simulink model "I2S"  (R2023b)
settings: Solver=VariableStepAuto  StartTime=0.0  StopTime=1  RelTol=1e-3
values from neighbouring files (symbols this model uses):
  cnt1_LRCLK = 511    [DATA_GEN.m]
  cnt2_SCLK = 7    [DATA_GEN.m]
libraries: hdlsllib x8
settings Model: Creator=31651  LastModifiedBy=31651

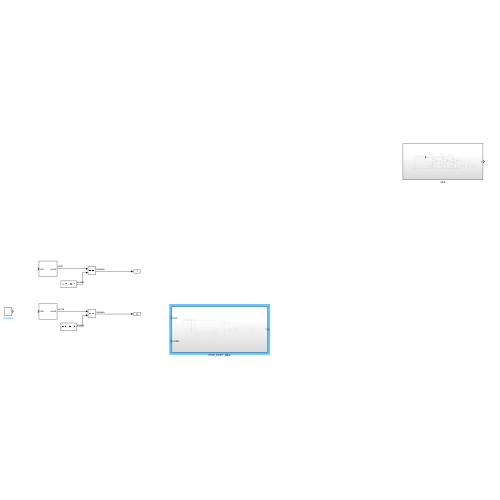
[thumbnail: Simulink's stored preview of the top-level diagram]
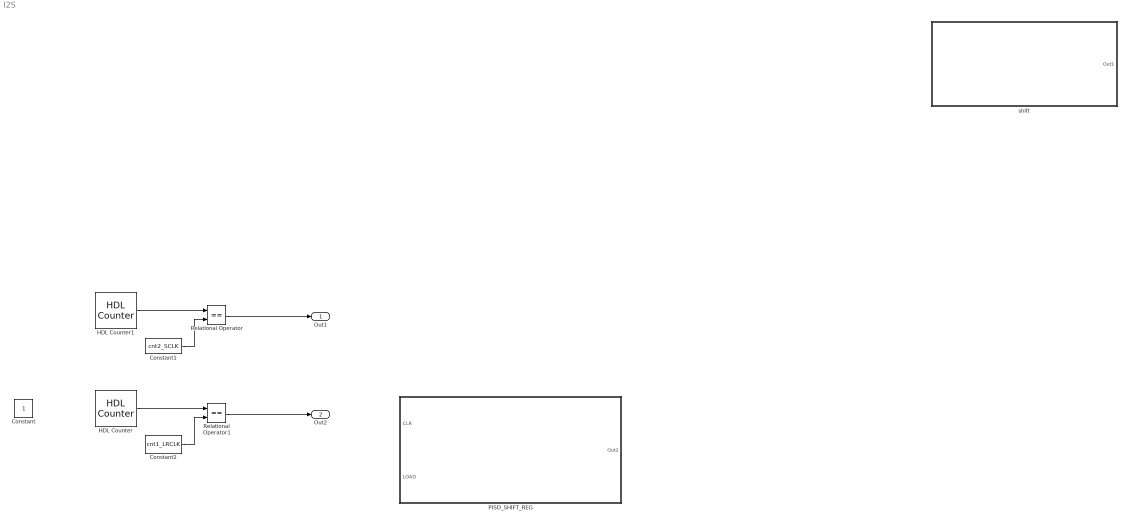
== system I2S ==
  Constant : Constant  OutDataTypeStr=boolean  SampleTime=1
  Constant1 : Constant  Value=cnt2_SCLK
  Constant2 : Constant  Value=cnt1_LRCLK
  HDL Counter : hdlsllib/Sources/HDL Counter  CountType=Count limited  CountInit=0  CountStep=1  CountMax=cnt1_LRCLK  CountFromType=Initial value  CountFrom=0  CountResetPort=off  CountLoadPort=off  CountEnbPort=on  CountDirPort=off  CountHitOutputPort=off  CountDataType=Unsigned  CountWordLen=16  CountFracLen=0  CountSampTime=1
  HDL Counter1 : hdlsllib/Sources/HDL Counter  CountType=Count limited  CountInit=0  CountStep=1  CountMax=cnt2_SCLK  CountFromType=Initial value  CountFrom=0  CountResetPort=off  CountLoadPort=off  CountEnbPort=on  CountDirPort=off  CountHitOutputPort=off  CountDataType=Unsigned  CountWordLen=8  CountFracLen=0  CountSampTime=1
  PISO_SHIFT_REG : Subsystem
  Relational Operator : RelationalOperator  Operator===  OutDataTypeStr=boolean  InputSameDT=off
  Relational Operator1 : RelationalOperator  Operator===  OutDataTypeStr=boolean  InputSameDT=off
  shift : Subsystem
  Out1 : Outport  VectorParamsAs1DForOutWhenUnconnected=off
  Out2 : Outport  Port=2  VectorParamsAs1DForOutWhenUnconnected=off
  wires:
  HDL Counter1/1 -> Relational Operator/1
  Constant1/1 -> Relational Operator/2
  Constant2/1 -> Relational Operator1/2
  HDL Counter/1 -> Relational Operator1/1
  Relational Operator/1 -> Out1/1
  Relational Operator1/1 -> Out2/1

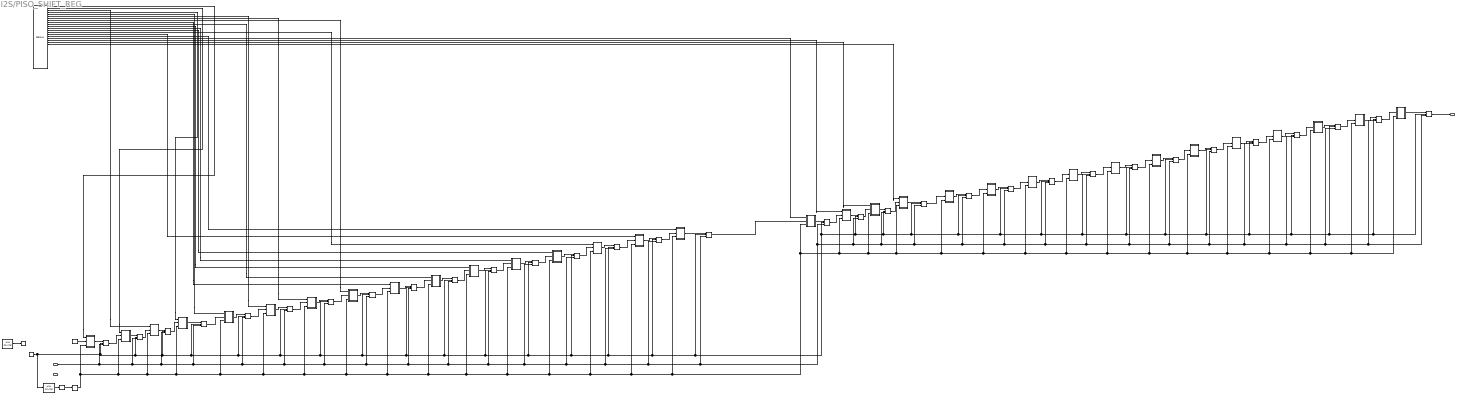
== system I2S/PISO_SHIFT_REG ==
  note: LOAD=0写入数据
      | LOAD=1 移位
  CLR : Inport
  LOAD : Inport  Port=2
  CLK : Constant  OutDataTypeStr=boolean  SampleTime=1/1000
  Compare To Constant : hdlsllib/Logic and Bit Operations/Compare To Constant  relop=>=  const=50  OutDataTypeStr=boolean
  Compare To Constant1 : hdlsllib/Logic and Bit Operations/Compare To Constant  relop=>=  const=10  OutDataTypeStr=boolean
  Constant5 : Constant  Value=0  OutDataTypeStr=boolean  SampleTime=1
  Delay{,1..15,17..24,26..33} (32 alike) : Delay  DelayLength=1  ExternalReset=Either  ShowEnablePort=on
      settings: InputPortMap=u0,e6,r5
  Delay16 : Delay  DelayLength=1  InitialCondition=0
  Demux : Demux  Outputs=32
      settings: DisplayOption=none
  HDL Counter : hdlsllib/Sources/HDL Counter  CountType=Count limited  CountInit=0  CountStep=1  CountMax=25  CountFromType=Initial value  CountFrom=0  CountResetPort=off  CountLoadPort=off  CountEnbPort=off  CountDirPort=off  CountHitOutputPort=off  CountDataType=Unsigned  CountWordLen=8  CountFracLen=0  CountSampTime=1
  HDL Counter1 : hdlsllib/Sources/HDL Counter  CountType=Count limited  CountInit=0  CountStep=1  CountMax=500  CountFromType=Initial value  CountFrom=0  CountResetPort=off  CountLoadPort=off  CountEnbPort=on  CountDirPort=off  CountHitOutputPort=off  CountDataType=Unsigned  CountWordLen=16  CountFracLen=0  CountSampTime=1
  MUX : Subsystem
  MUX1 : Subsystem
  MUX10 : Subsystem
  MUX11 : Subsystem
  MUX12 : Subsystem
  MUX13 : Subsystem
  MUX14 : Subsystem
  MUX15 : Subsystem
  MUX16 : Subsystem
  MUX17 : Subsystem
  MUX18 : Subsystem
  MUX19 : Subsystem
  MUX2 : Subsystem
  MUX20 : Subsystem
  MUX21 : Subsystem
  MUX22 : Subsystem
  MUX23 : Subsystem
  MUX24 : Subsystem
  MUX25 : Subsystem
  MUX26 : Subsystem
  MUX27 : Subsystem
  MUX28 : Subsystem
  MUX29 : Subsystem
  MUX3 : Subsystem
  MUX30 : Subsystem
  MUX31 : Subsystem
  MUX4 : Subsystem
  MUX5 : Subsystem
  MUX6 : Subsystem
  MUX7 : Subsystem
  MUX8 : Subsystem
  MUX9 : Subsystem
  Out2 : Outport  VectorParamsAs1DForOutWhenUnconnected=off
  wires:
  MUX/1(Out1) -> Delay/1
  Demux/2 -> MUX1/1(In1)
  MUX1/1(Out1) -> Delay1/1
  Delay/1 -> MUX1/2(In2)
  MUX2/1(Out1) -> Delay2/1
  Demux/3 -> MUX2/1(In1)
  Delay1/1 -> MUX2/2(In2)
  Demux/4 -> MUX3/1(In1)
  Delay2/1 -> MUX3/2(In2)
  MUX3/1(Out1) -> Delay3/1
  Constant5/1 -> MUX/2(In2)
  Demux/1 -> MUX/1(In1)
  MUX4/1(Out1) -> Delay4/1
  MUX5/1(Out1) -> Delay5/1
  MUX6/1(Out1) -> Delay6/1
  Delay3/1 -> MUX4/2(In2)
  Delay4/1 -> MUX5/2(In2)
  Delay5/1 -> MUX6/2(In2)
  Delay8/1 -> MUX9/2(In2)
  Delay7/1 -> MUX8/2(In2)
  MUX8/1(Out1) -> Delay8/1
  MUX9/1(Out1) -> Delay9/1
  MUX7/1(Out1) -> Delay7/1
  Delay11/1 -> MUX12/2(In2)
  Delay10/1 -> MUX11/2(In2)
  MUX11/1(Out1) -> Delay11/1
  MUX12/1(Out1) -> Delay12/1
  MUX10/1(Out1) -> Delay10/1
  Delay14/1 -> MUX15/2(In2)
  Delay13/1 -> MUX14/2(In2)
  MUX14/1(Out1) -> Delay14/1
  MUX15/1(Out1) -> Delay15/1
  MUX13/1(Out1) -> Delay13/1
  Delay6/1 -> MUX7/2(In2)
  Delay9/1 -> MUX10/2(In2)
  Delay12/1 -> MUX13/2(In2)
  Demux/5 -> MUX4/1(In1)
  Demux/6 -> MUX5/1(In1)
  Demux/7 -> MUX6/1(In1)
  Demux/8 -> MUX7/1(In1)
  Demux/9 -> MUX8/1(In1)
  Demux/10 -> MUX9/1(In1)
  Demux/11 -> MUX10/1(In1)
  Demux/12 -> MUX11/1(In1)
  Demux/13 -> MUX12/1(In1)
  Demux/14 -> MUX13/1(In1)
  Demux/15 -> MUX14/1(In1)
  Demux/16 -> MUX15/1(In1)
  HDL Counter/1 -> Compare To Constant/1
  Compare To Constant1/1 -> Delay16/1
  HDL Counter1/1 -> Compare To Constant1/1
  ? -> MUX21/1(In1)
  CLK/1 -> HDL Counter1/1, Delay1/2, Delay2/2, Delay8/2, Delay10/2, Delay11/2, Delay12/2, Delay13/2, Delay14/2, Delay15/2, Delay17/2, Delay18/2, Delay26/2, Delay32/2, Delay19/2, Delay20/2, Delay21/2, Delay22/2, Delay23/2, Delay24/2, Delay33/2, Delay31/2, Delay30/2, Delay29/2, Delay28/2, Delay27/2, Delay9/2, Delay7/2, Delay6/2, Delay5/2, Delay4/2, Delay3/2, Delay/2
  ? -> MUX29/1(In1)
  ? -> MUX19/1(In1)
  ? -> MUX18/1(In1)
  Delay26/1 -> MUX25/2(In2)
  MUX25/1(Out1) -> Delay27/1
  Delay16/1 -> MUX/3(SEL), MUX1/3(SEL), MUX4/3(SEL), MUX5/3(SEL), MUX6/3(SEL), MUX7/3(SEL), MUX8/3(SEL), MUX9/3(SEL), MUX10/3(SEL), MUX11/3(SEL), MUX12/3(SEL), MUX13/3(SEL), MUX14/3(SEL), MUX15/3(SEL), MUX16/3(SEL), MUX17/3(SEL), MUX26/3(SEL), MUX27/3(SEL), MUX28/3(SEL), MUX29/3(SEL), MUX30/3(SEL), MUX31/3(SEL), MUX18/3(SEL), MUX19/3(SEL), MUX20/3(SEL), MUX21/3(SEL), MUX22/3(SEL), MUX23/3(SEL), MUX25/3(SEL), MUX24/3(SEL), MUX3/3(SEL), MUX2/3(SEL)
  MUX31/1(Out1) -> Delay33/1
  MUX29/1(Out1) -> Delay31/1
  MUX30/1(Out1) -> Delay32/1
  Delay31/1 -> MUX30/2(In2)
  Delay32/1 -> MUX31/2(In2)
  MUX17/1(Out1) -> Delay18/1
  Delay17/1 -> MUX17/2(In2)
  MUX16/1(Out1) -> Delay17/1
  ? -> MUX28/1(In1)
  Delay29/1 -> MUX28/2(In2)
  Delay28/1 -> MUX27/2(In2)
  ? -> MUX27/1(In1)
  MUX27/1(Out1) -> Delay29/1
  Delay21/1 -> MUX21/2(In2)
  MUX20/1(Out1) -> Delay21/1
  ? -> MUX31/1(In1)
  Delay24/1 -> Out2/1
  Demux/20 -> MUX25/1(In1)
  CLR/1 -> Delay/3, Delay24/3, Delay23/3, Delay22/3, Delay21/3, Delay20/3, Delay19/3, Delay33/3, Delay32/3, Delay31/3, Delay30/3, Delay29/3, Delay28/3, Delay27/3, Delay26/3, Delay18/3, Delay17/3, Delay15/3, Delay14/3, Delay13/3, Delay12/3, Delay11/3, Delay10/3, Delay9/3, Delay8/3, Delay7/3, Delay6/3, Delay5/3, Delay4/3, Delay3/3, Delay2/3, Delay1/3
  ? -> MUX20/1(In1)
  Demux/18 -> MUX17/1(In1)
  Demux/17 -> MUX16/1(In1)
  Delay18/1 -> MUX24/2(In2)
  ? -> MUX26/1(In1)
  ? -> MUX22/1(In1)
  ? -> MUX30/1(In1)
  Delay27/1 -> MUX26/2(In2)
  MUX26/1(Out1) -> Delay28/1
  Delay20/1 -> MUX20/2(In2)
  MUX18/1(Out1) -> Delay19/1
  Delay19/1 -> MUX19/2(In2)
  MUX28/1(Out1) -> Delay30/1
  MUX23/1(Out1) -> Delay24/1
  Delay15/1 -> MUX16/2(In2)
  Delay33/1 -> MUX18/2(In2)
  Delay22/1 -> MUX22/2(In2)
  Delay23/1 -> MUX23/2(In2)
  ? -> MUX23/1(In1)
  MUX21/1(Out1) -> Delay22/1
  MUX24/1(Out1) -> Delay26/1
  Delay30/1 -> MUX29/2(In2)
  MUX19/1(Out1) -> Delay20/1
  MUX22/1(Out1) -> Delay23/1
  Demux/19 -> MUX24/1(In1)

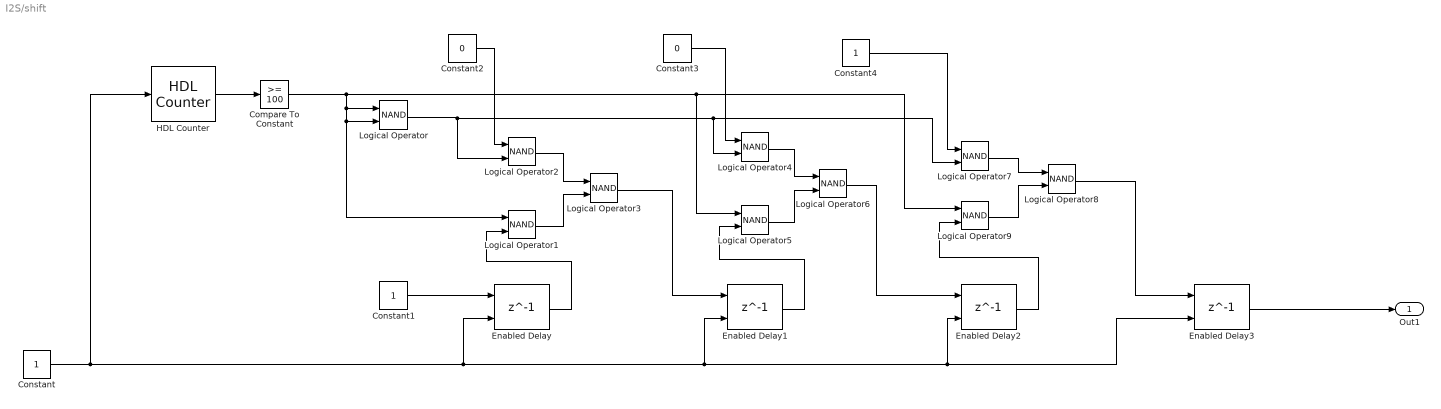
== system I2S/shift ==
  Compare To Constant : hdlsllib/Logic and Bit Operations/Compare To Constant  relop=>=  const=100  OutDataTypeStr=boolean
  Constant : Constant  OutDataTypeStr=boolean  SampleTime=1
  Constant1 : Constant  OutDataTypeStr=boolean  SampleTime=1
  Constant2 : Constant  Value=0  OutDataTypeStr=boolean  SampleTime=1
  Constant3 : Constant  Value=0  OutDataTypeStr=boolean  SampleTime=1
  Constant4 : Constant  OutDataTypeStr=boolean  SampleTime=1
  Enabled Delay{,1..3} (4 alike) : Delay  DelayLength=1  ShowEnablePort=on
      settings: InputPortMap=u0,e6
  HDL Counter : hdlsllib/Sources/HDL Counter  CountType=Count limited  CountInit=0  CountStep=1  CountMax=1000  CountFromType=Initial value  CountFrom=0  CountResetPort=off  CountLoadPort=off  CountEnbPort=on  CountDirPort=off  CountHitOutputPort=off  CountDataType=Unsigned  CountWordLen=16  CountFracLen=0  CountSampTime=1
  Logical Operator{,1..9} (10 alike) : Logic  Operator=NAND  AllPortsSameDT=off  OutDataTypeStr=boolean
  Out1 : Outport  VectorParamsAs1DForOutWhenUnconnected=off
  wires:
  Logical Operator1/1 -> Logical Operator3/2
  Logical Operator2/1 -> Logical Operator3/1
  Logical Operator/1 -> Logical Operator2/2, Logical Operator7/2, Logical Operator4/2
  Enabled Delay/1 -> Logical Operator1/2
  Compare To Constant/1 -> Logical Operator9/1, Logical Operator5/1, Logical Operator1/1, Logical Operator/2, Logical Operator/1
  Logical Operator5/1 -> Logical Operator6/2
  Logical Operator4/1 -> Logical Operator6/1
  Logical Operator3/1 -> Enabled Delay1/1
  Enabled Delay1/1 -> Logical Operator5/2
  Logical Operator7/1 -> Logical Operator8/1
  Logical Operator9/1 -> Logical Operator8/2
  Enabled Delay2/1 -> Logical Operator9/2
  Logical Operator6/1 -> Enabled Delay2/1
  Logical Operator8/1 -> Enabled Delay3/1
  Constant/1 -> HDL Counter/1, Enabled Delay/2, Enabled Delay1/2, Enabled Delay3/2, Enabled Delay2/2
  Constant2/1 -> Logical Operator2/1
  Constant3/1 -> Logical Operator4/1
  Constant4/1 -> Logical Operator7/1
  Enabled Delay3/1 -> Out1/1
  Constant1/1 -> Enabled Delay/1
  HDL Counter/1 -> Compare To Constant/1

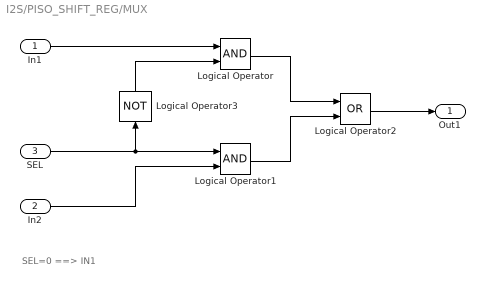
== system I2S/PISO_SHIFT_REG/MUX ==
  note: SEL=0 ==> IN1
  In1 : Inport
  In2 : Inport  Port=2
  SEL : Inport  Port=3  OutDataTypeStr=boolean
  Logical Operator : Logic  AllPortsSameDT=off  OutDataTypeStr=boolean
  Logical Operator1 : Logic  AllPortsSameDT=off  OutDataTypeStr=boolean
  Logical Operator2 : Logic  Operator=OR  AllPortsSameDT=off  OutDataTypeStr=boolean
  Logical Operator3 : Logic  Operator=NOT  AllPortsSameDT=off  OutDataTypeStr=boolean
  Out1 : Outport  VectorParamsAs1DForOutWhenUnconnected=off
  wires:
  In1/1 -> Logical Operator/1
  SEL/1 -> Logical Operator3/1, Logical Operator1/1
  Logical Operator3/1 -> Logical Operator/2
  Logical Operator1/1 -> Logical Operator2/2
  Logical Operator/1 -> Logical Operator2/1
  Logical Operator2/1 -> Out1/1
  In2/1 -> Logical Operator1/2

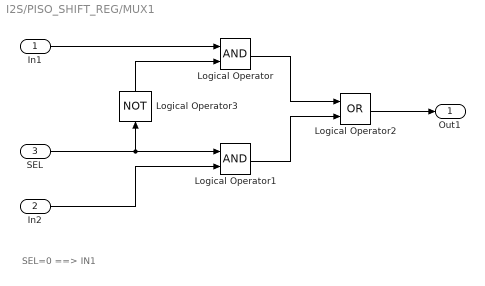
== system I2S/PISO_SHIFT_REG/MUX1 ==
  note: SEL=0 ==> IN1
  In1 : Inport
  In2 : Inport  Port=2
  SEL : Inport  Port=3  OutDataTypeStr=boolean
  Logical Operator : Logic  AllPortsSameDT=off  OutDataTypeStr=boolean
  Logical Operator1 : Logic  AllPortsSameDT=off  OutDataTypeStr=boolean
  Logical Operator2 : Logic  Operator=OR  AllPortsSameDT=off  OutDataTypeStr=boolean
  Logical Operator3 : Logic  Operator=NOT  AllPortsSameDT=off  OutDataTypeStr=boolean
  Out1 : Outport  VectorParamsAs1DForOutWhenUnconnected=off
  wires:
  In1/1 -> Logical Operator/1
  SEL/1 -> Logical Operator3/1, Logical Operator1/1
  Logical Operator3/1 -> Logical Operator/2
  Logical Operator1/1 -> Logical Operator2/2
  Logical Operator/1 -> Logical Operator2/1
  Logical Operator2/1 -> Out1/1
  In2/1 -> Logical Operator1/2

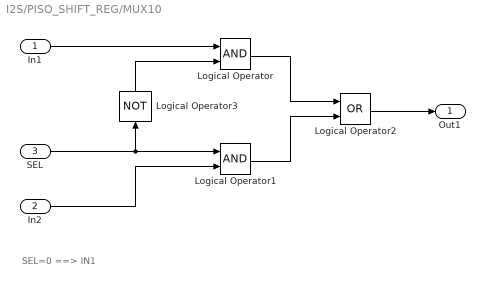
== system I2S/PISO_SHIFT_REG/MUX10 ==
  note: SEL=0 ==> IN1
  In1 : Inport
  In2 : Inport  Port=2
  SEL : Inport  Port=3  OutDataTypeStr=boolean
  Logical Operator : Logic  AllPortsSameDT=off  OutDataTypeStr=boolean
  Logical Operator1 : Logic  AllPortsSameDT=off  OutDataTypeStr=boolean
  Logical Operator2 : Logic  Operator=OR  AllPortsSameDT=off  OutDataTypeStr=boolean
  Logical Operator3 : Logic  Operator=NOT  AllPortsSameDT=off  OutDataTypeStr=boolean
  Out1 : Outport  VectorParamsAs1DForOutWhenUnconnected=off
  wires:
  In1/1 -> Logical Operator/1
  SEL/1 -> Logical Operator3/1, Logical Operator1/1
  Logical Operator3/1 -> Logical Operator/2
  Logical Operator1/1 -> Logical Operator2/2
  Logical Operator/1 -> Logical Operator2/1
  Logical Operator2/1 -> Out1/1
  In2/1 -> Logical Operator1/2

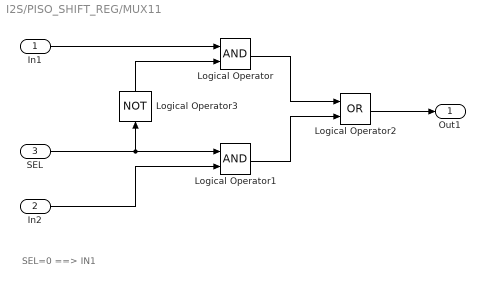
== system I2S/PISO_SHIFT_REG/MUX11 ==
  note: SEL=0 ==> IN1
  In1 : Inport
  In2 : Inport  Port=2
  SEL : Inport  Port=3  OutDataTypeStr=boolean
  Logical Operator : Logic  AllPortsSameDT=off  OutDataTypeStr=boolean
  Logical Operator1 : Logic  AllPortsSameDT=off  OutDataTypeStr=boolean
  Logical Operator2 : Logic  Operator=OR  AllPortsSameDT=off  OutDataTypeStr=boolean
  Logical Operator3 : Logic  Operator=NOT  AllPortsSameDT=off  OutDataTypeStr=boolean
  Out1 : Outport  VectorParamsAs1DForOutWhenUnconnected=off
  wires:
  In1/1 -> Logical Operator/1
  SEL/1 -> Logical Operator3/1, Logical Operator1/1
  Logical Operator3/1 -> Logical Operator/2
  Logical Operator1/1 -> Logical Operator2/2
  Logical Operator/1 -> Logical Operator2/1
  Logical Operator2/1 -> Out1/1
  In2/1 -> Logical Operator1/2

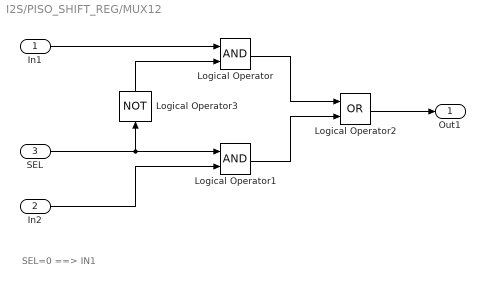
== system I2S/PISO_SHIFT_REG/MUX12 ==
  note: SEL=0 ==> IN1
  In1 : Inport
  In2 : Inport  Port=2
  SEL : Inport  Port=3  OutDataTypeStr=boolean
  Logical Operator : Logic  AllPortsSameDT=off  OutDataTypeStr=boolean
  Logical Operator1 : Logic  AllPortsSameDT=off  OutDataTypeStr=boolean
  Logical Operator2 : Logic  Operator=OR  AllPortsSameDT=off  OutDataTypeStr=boolean
  Logical Operator3 : Logic  Operator=NOT  AllPortsSameDT=off  OutDataTypeStr=boolean
  Out1 : Outport  VectorParamsAs1DForOutWhenUnconnected=off
  wires:
  In1/1 -> Logical Operator/1
  SEL/1 -> Logical Operator3/1, Logical Operator1/1
  Logical Operator3/1 -> Logical Operator/2
  Logical Operator1/1 -> Logical Operator2/2
  Logical Operator/1 -> Logical Operator2/1
  Logical Operator2/1 -> Out1/1
  In2/1 -> Logical Operator1/2

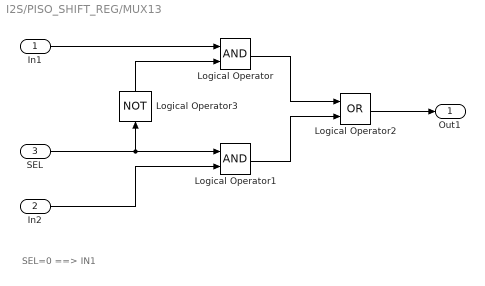
== system I2S/PISO_SHIFT_REG/MUX13 ==
  note: SEL=0 ==> IN1
  In1 : Inport
  In2 : Inport  Port=2
  SEL : Inport  Port=3  OutDataTypeStr=boolean
  Logical Operator : Logic  AllPortsSameDT=off  OutDataTypeStr=boolean
  Logical Operator1 : Logic  AllPortsSameDT=off  OutDataTypeStr=boolean
  Logical Operator2 : Logic  Operator=OR  AllPortsSameDT=off  OutDataTypeStr=boolean
  Logical Operator3 : Logic  Operator=NOT  AllPortsSameDT=off  OutDataTypeStr=boolean
  Out1 : Outport  VectorParamsAs1DForOutWhenUnconnected=off
  wires:
  In1/1 -> Logical Operator/1
  SEL/1 -> Logical Operator3/1, Logical Operator1/1
  Logical Operator3/1 -> Logical Operator/2
  Logical Operator1/1 -> Logical Operator2/2
  Logical Operator/1 -> Logical Operator2/1
  Logical Operator2/1 -> Out1/1
  In2/1 -> Logical Operator1/2

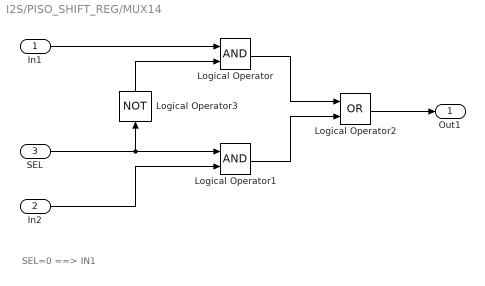
== system I2S/PISO_SHIFT_REG/MUX14 ==
  note: SEL=0 ==> IN1
  In1 : Inport
  In2 : Inport  Port=2
  SEL : Inport  Port=3  OutDataTypeStr=boolean
  Logical Operator : Logic  AllPortsSameDT=off  OutDataTypeStr=boolean
  Logical Operator1 : Logic  AllPortsSameDT=off  OutDataTypeStr=boolean
  Logical Operator2 : Logic  Operator=OR  AllPortsSameDT=off  OutDataTypeStr=boolean
  Logical Operator3 : Logic  Operator=NOT  AllPortsSameDT=off  OutDataTypeStr=boolean
  Out1 : Outport  VectorParamsAs1DForOutWhenUnconnected=off
  wires:
  In1/1 -> Logical Operator/1
  SEL/1 -> Logical Operator3/1, Logical Operator1/1
  Logical Operator3/1 -> Logical Operator/2
  Logical Operator1/1 -> Logical Operator2/2
  Logical Operator/1 -> Logical Operator2/1
  Logical Operator2/1 -> Out1/1
  In2/1 -> Logical Operator1/2

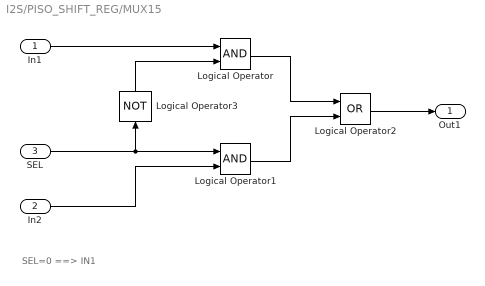
== system I2S/PISO_SHIFT_REG/MUX15 ==
  note: SEL=0 ==> IN1
  In1 : Inport
  In2 : Inport  Port=2
  SEL : Inport  Port=3  OutDataTypeStr=boolean
  Logical Operator : Logic  AllPortsSameDT=off  OutDataTypeStr=boolean
  Logical Operator1 : Logic  AllPortsSameDT=off  OutDataTypeStr=boolean
  Logical Operator2 : Logic  Operator=OR  AllPortsSameDT=off  OutDataTypeStr=boolean
  Logical Operator3 : Logic  Operator=NOT  AllPortsSameDT=off  OutDataTypeStr=boolean
  Out1 : Outport  VectorParamsAs1DForOutWhenUnconnected=off
  wires:
  In1/1 -> Logical Operator/1
  SEL/1 -> Logical Operator3/1, Logical Operator1/1
  Logical Operator3/1 -> Logical Operator/2
  Logical Operator1/1 -> Logical Operator2/2
  Logical Operator/1 -> Logical Operator2/1
  Logical Operator2/1 -> Out1/1
  In2/1 -> Logical Operator1/2

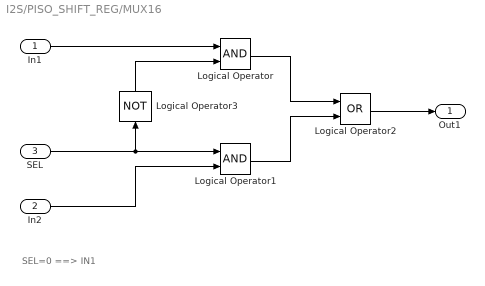
== system I2S/PISO_SHIFT_REG/MUX16 ==
  note: SEL=0 ==> IN1
  In1 : Inport
  In2 : Inport  Port=2
  SEL : Inport  Port=3  OutDataTypeStr=boolean
  Logical Operator : Logic  AllPortsSameDT=off  OutDataTypeStr=boolean
  Logical Operator1 : Logic  AllPortsSameDT=off  OutDataTypeStr=boolean
  Logical Operator2 : Logic  Operator=OR  AllPortsSameDT=off  OutDataTypeStr=boolean
  Logical Operator3 : Logic  Operator=NOT  AllPortsSameDT=off  OutDataTypeStr=boolean
  Out1 : Outport  VectorParamsAs1DForOutWhenUnconnected=off
  wires:
  In1/1 -> Logical Operator/1
  SEL/1 -> Logical Operator3/1, Logical Operator1/1
  Logical Operator3/1 -> Logical Operator/2
  Logical Operator1/1 -> Logical Operator2/2
  Logical Operator/1 -> Logical Operator2/1
  Logical Operator2/1 -> Out1/1
  In2/1 -> Logical Operator1/2

== system I2S/PISO_SHIFT_REG/MUX17 ==
  note: SEL=0 ==> IN1
  In1 : Inport
  In2 : Inport  Port=2
  SEL : Inport  Port=3  OutDataTypeStr=boolean
  Logical Operator : Logic  AllPortsSameDT=off  OutDataTypeStr=boolean
  Logical Operator1 : Logic  AllPortsSameDT=off  OutDataTypeStr=boolean
  Logical Operator2 : Logic  Operator=OR  AllPortsSameDT=off  OutDataTypeStr=boolean
  Logical Operator3 : Logic  Operator=NOT  AllPortsSameDT=off  OutDataTypeStr=boolean
  Out1 : Outport  VectorParamsAs1DForOutWhenUnconnected=off
  wires:
  In1/1 -> Logical Operator/1
  SEL/1 -> Logical Operator3/1, Logical Operator1/1
  Logical Operator3/1 -> Logical Operator/2
  Logical Operator1/1 -> Logical Operator2/2
  Logical Operator/1 -> Logical Operator2/1
  Logical Operator2/1 -> Out1/1
  In2/1 -> Logical Operator1/2

== system I2S/PISO_SHIFT_REG/MUX18 ==
  note: SEL=0 ==> IN1
  In1 : Inport
  In2 : Inport  Port=2
  SEL : Inport  Port=3  OutDataTypeStr=boolean
  Logical Operator : Logic  AllPortsSameDT=off  OutDataTypeStr=boolean
  Logical Operator1 : Logic  AllPortsSameDT=off  OutDataTypeStr=boolean
  Logical Operator2 : Logic  Operator=OR  AllPortsSameDT=off  OutDataTypeStr=boolean
  Logical Operator3 : Logic  Operator=NOT  AllPortsSameDT=off  OutDataTypeStr=boolean
  Out1 : Outport  VectorParamsAs1DForOutWhenUnconnected=off
  wires:
  In1/1 -> Logical Operator/1
  SEL/1 -> Logical Operator3/1, Logical Operator1/1
  Logical Operator3/1 -> Logical Operator/2
  Logical Operator1/1 -> Logical Operator2/2
  Logical Operator/1 -> Logical Operator2/1
  Logical Operator2/1 -> Out1/1
  In2/1 -> Logical Operator1/2

== system I2S/PISO_SHIFT_REG/MUX19 ==
  note: SEL=0 ==> IN1
  In1 : Inport
  In2 : Inport  Port=2
  SEL : Inport  Port=3  OutDataTypeStr=boolean
  Logical Operator : Logic  AllPortsSameDT=off  OutDataTypeStr=boolean
  Logical Operator1 : Logic  AllPortsSameDT=off  OutDataTypeStr=boolean
  Logical Operator2 : Logic  Operator=OR  AllPortsSameDT=off  OutDataTypeStr=boolean
  Logical Operator3 : Logic  Operator=NOT  AllPortsSameDT=off  OutDataTypeStr=boolean
  Out1 : Outport  VectorParamsAs1DForOutWhenUnconnected=off
  wires:
  In1/1 -> Logical Operator/1
  SEL/1 -> Logical Operator3/1, Logical Operator1/1
  Logical Operator3/1 -> Logical Operator/2
  Logical Operator1/1 -> Logical Operator2/2
  Logical Operator/1 -> Logical Operator2/1
  Logical Operator2/1 -> Out1/1
  In2/1 -> Logical Operator1/2

== system I2S/PISO_SHIFT_REG/MUX2 ==
  note: SEL=0 ==> IN1
  In1 : Inport
  In2 : Inport  Port=2
  SEL : Inport  Port=3  OutDataTypeStr=boolean
  Logical Operator : Logic  AllPortsSameDT=off  OutDataTypeStr=boolean
  Logical Operator1 : Logic  AllPortsSameDT=off  OutDataTypeStr=boolean
  Logical Operator2 : Logic  Operator=OR  AllPortsSameDT=off  OutDataTypeStr=boolean
  Logical Operator3 : Logic  Operator=NOT  AllPortsSameDT=off  OutDataTypeStr=boolean
  Out1 : Outport  VectorParamsAs1DForOutWhenUnconnected=off
  wires:
  In1/1 -> Logical Operator/1
  SEL/1 -> Logical Operator3/1, Logical Operator1/1
  Logical Operator3/1 -> Logical Operator/2
  Logical Operator1/1 -> Logical Operator2/2
  Logical Operator/1 -> Logical Operator2/1
  Logical Operator2/1 -> Out1/1
  In2/1 -> Logical Operator1/2

== system I2S/PISO_SHIFT_REG/MUX20 ==
  note: SEL=0 ==> IN1
  In1 : Inport
  In2 : Inport  Port=2
  SEL : Inport  Port=3  OutDataTypeStr=boolean
  Logical Operator : Logic  AllPortsSameDT=off  OutDataTypeStr=boolean
  Logical Operator1 : Logic  AllPortsSameDT=off  OutDataTypeStr=boolean
  Logical Operator2 : Logic  Operator=OR  AllPortsSameDT=off  OutDataTypeStr=boolean
  Logical Operator3 : Logic  Operator=NOT  AllPortsSameDT=off  OutDataTypeStr=boolean
  Out1 : Outport  VectorParamsAs1DForOutWhenUnconnected=off
  wires:
  In1/1 -> Logical Operator/1
  SEL/1 -> Logical Operator3/1, Logical Operator1/1
  Logical Operator3/1 -> Logical Operator/2
  Logical Operator1/1 -> Logical Operator2/2
  Logical Operator/1 -> Logical Operator2/1
  Logical Operator2/1 -> Out1/1
  In2/1 -> Logical Operator1/2

== system I2S/PISO_SHIFT_REG/MUX21 ==
  note: SEL=0 ==> IN1
  In1 : Inport
  In2 : Inport  Port=2
  SEL : Inport  Port=3  OutDataTypeStr=boolean
  Logical Operator : Logic  AllPortsSameDT=off  OutDataTypeStr=boolean
  Logical Operator1 : Logic  AllPortsSameDT=off  OutDataTypeStr=boolean
  Logical Operator2 : Logic  Operator=OR  AllPortsSameDT=off  OutDataTypeStr=boolean
  Logical Operator3 : Logic  Operator=NOT  AllPortsSameDT=off  OutDataTypeStr=boolean
  Out1 : Outport  VectorParamsAs1DForOutWhenUnconnected=off
  wires:
  In1/1 -> Logical Operator/1
  SEL/1 -> Logical Operator3/1, Logical Operator1/1
  Logical Operator3/1 -> Logical Operator/2
  Logical Operator1/1 -> Logical Operator2/2
  Logical Operator/1 -> Logical Operator2/1
  Logical Operator2/1 -> Out1/1
  In2/1 -> Logical Operator1/2

== system I2S/PISO_SHIFT_REG/MUX22 ==
  note: SEL=0 ==> IN1
  In1 : Inport
  In2 : Inport  Port=2
  SEL : Inport  Port=3  OutDataTypeStr=boolean
  Logical Operator : Logic  AllPortsSameDT=off  OutDataTypeStr=boolean
  Logical Operator1 : Logic  AllPortsSameDT=off  OutDataTypeStr=boolean
  Logical Operator2 : Logic  Operator=OR  AllPortsSameDT=off  OutDataTypeStr=boolean
  Logical Operator3 : Logic  Operator=NOT  AllPortsSameDT=off  OutDataTypeStr=boolean
  Out1 : Outport  VectorParamsAs1DForOutWhenUnconnected=off
  wires:
  In1/1 -> Logical Operator/1
  SEL/1 -> Logical Operator3/1, Logical Operator1/1
  Logical Operator3/1 -> Logical Operator/2
  Logical Operator1/1 -> Logical Operator2/2
  Logical Operator/1 -> Logical Operator2/1
  Logical Operator2/1 -> Out1/1
  In2/1 -> Logical Operator1/2

== system I2S/PISO_SHIFT_REG/MUX23 ==
  note: SEL=0 ==> IN1
  In1 : Inport
  In2 : Inport  Port=2
  SEL : Inport  Port=3  OutDataTypeStr=boolean
  Logical Operator : Logic  AllPortsSameDT=off  OutDataTypeStr=boolean
  Logical Operator1 : Logic  AllPortsSameDT=off  OutDataTypeStr=boolean
  Logical Operator2 : Logic  Operator=OR  AllPortsSameDT=off  OutDataTypeStr=boolean
  Logical Operator3 : Logic  Operator=NOT  AllPortsSameDT=off  OutDataTypeStr=boolean
  Out1 : Outport  VectorParamsAs1DForOutWhenUnconnected=off
  wires:
  In1/1 -> Logical Operator/1
  SEL/1 -> Logical Operator3/1, Logical Operator1/1
  Logical Operator3/1 -> Logical Operator/2
  Logical Operator1/1 -> Logical Operator2/2
  Logical Operator/1 -> Logical Operator2/1
  Logical Operator2/1 -> Out1/1
  In2/1 -> Logical Operator1/2

== system I2S/PISO_SHIFT_REG/MUX24 ==
  note: SEL=0 ==> IN1
  In1 : Inport
  In2 : Inport  Port=2
  SEL : Inport  Port=3  OutDataTypeStr=boolean
  Logical Operator : Logic  AllPortsSameDT=off  OutDataTypeStr=boolean
  Logical Operator1 : Logic  AllPortsSameDT=off  OutDataTypeStr=boolean
  Logical Operator2 : Logic  Operator=OR  AllPortsSameDT=off  OutDataTypeStr=boolean
  Logical Operator3 : Logic  Operator=NOT  AllPortsSameDT=off  OutDataTypeStr=boolean
  Out1 : Outport  VectorParamsAs1DForOutWhenUnconnected=off
  wires:
  In1/1 -> Logical Operator/1
  SEL/1 -> Logical Operator3/1, Logical Operator1/1
  Logical Operator3/1 -> Logical Operator/2
  Logical Operator1/1 -> Logical Operator2/2
  Logical Operator/1 -> Logical Operator2/1
  Logical Operator2/1 -> Out1/1
  In2/1 -> Logical Operator1/2

== system I2S/PISO_SHIFT_REG/MUX25 ==
  note: SEL=0 ==> IN1
  In1 : Inport
  In2 : Inport  Port=2
  SEL : Inport  Port=3  OutDataTypeStr=boolean
  Logical Operator : Logic  AllPortsSameDT=off  OutDataTypeStr=boolean
  Logical Operator1 : Logic  AllPortsSameDT=off  OutDataTypeStr=boolean
  Logical Operator2 : Logic  Operator=OR  AllPortsSameDT=off  OutDataTypeStr=boolean
  Logical Operator3 : Logic  Operator=NOT  AllPortsSameDT=off  OutDataTypeStr=boolean
  Out1 : Outport  VectorParamsAs1DForOutWhenUnconnected=off
  wires:
  In1/1 -> Logical Operator/1
  SEL/1 -> Logical Operator3/1, Logical Operator1/1
  Logical Operator3/1 -> Logical Operator/2
  Logical Operator1/1 -> Logical Operator2/2
  Logical Operator/1 -> Logical Operator2/1
  Logical Operator2/1 -> Out1/1
  In2/1 -> Logical Operator1/2

== system I2S/PISO_SHIFT_REG/MUX26 ==
  note: SEL=0 ==> IN1
  In1 : Inport
  In2 : Inport  Port=2
  SEL : Inport  Port=3  OutDataTypeStr=boolean
  Logical Operator : Logic  AllPortsSameDT=off  OutDataTypeStr=boolean
  Logical Operator1 : Logic  AllPortsSameDT=off  OutDataTypeStr=boolean
  Logical Operator2 : Logic  Operator=OR  AllPortsSameDT=off  OutDataTypeStr=boolean
  Logical Operator3 : Logic  Operator=NOT  AllPortsSameDT=off  OutDataTypeStr=boolean
  Out1 : Outport  VectorParamsAs1DForOutWhenUnconnected=off
  wires:
  In1/1 -> Logical Operator/1
  SEL/1 -> Logical Operator3/1, Logical Operator1/1
  Logical Operator3/1 -> Logical Operator/2
  Logical Operator1/1 -> Logical Operator2/2
  Logical Operator/1 -> Logical Operator2/1
  Logical Operator2/1 -> Out1/1
  In2/1 -> Logical Operator1/2

== system I2S/PISO_SHIFT_REG/MUX27 ==
  note: SEL=0 ==> IN1
  In1 : Inport
  In2 : Inport  Port=2
  SEL : Inport  Port=3  OutDataTypeStr=boolean
  Logical Operator : Logic  AllPortsSameDT=off  OutDataTypeStr=boolean
  Logical Operator1 : Logic  AllPortsSameDT=off  OutDataTypeStr=boolean
  Logical Operator2 : Logic  Operator=OR  AllPortsSameDT=off  OutDataTypeStr=boolean
  Logical Operator3 : Logic  Operator=NOT  AllPortsSameDT=off  OutDataTypeStr=boolean
  Out1 : Outport  VectorParamsAs1DForOutWhenUnconnected=off
  wires:
  In1/1 -> Logical Operator/1
  SEL/1 -> Logical Operator3/1, Logical Operator1/1
  Logical Operator3/1 -> Logical Operator/2
  Logical Operator1/1 -> Logical Operator2/2
  Logical Operator/1 -> Logical Operator2/1
  Logical Operator2/1 -> Out1/1
  In2/1 -> Logical Operator1/2

== system I2S/PISO_SHIFT_REG/MUX28 ==
  note: SEL=0 ==> IN1
  In1 : Inport
  In2 : Inport  Port=2
  SEL : Inport  Port=3  OutDataTypeStr=boolean
  Logical Operator : Logic  AllPortsSameDT=off  OutDataTypeStr=boolean
  Logical Operator1 : Logic  AllPortsSameDT=off  OutDataTypeStr=boolean
  Logical Operator2 : Logic  Operator=OR  AllPortsSameDT=off  OutDataTypeStr=boolean
  Logical Operator3 : Logic  Operator=NOT  AllPortsSameDT=off  OutDataTypeStr=boolean
  Out1 : Outport  VectorParamsAs1DForOutWhenUnconnected=off
  wires:
  In1/1 -> Logical Operator/1
  SEL/1 -> Logical Operator3/1, Logical Operator1/1
  Logical Operator3/1 -> Logical Operator/2
  Logical Operator1/1 -> Logical Operator2/2
  Logical Operator/1 -> Logical Operator2/1
  Logical Operator2/1 -> Out1/1
  In2/1 -> Logical Operator1/2

== system I2S/PISO_SHIFT_REG/MUX29 ==
  note: SEL=0 ==> IN1
  In1 : Inport
  In2 : Inport  Port=2
  SEL : Inport  Port=3  OutDataTypeStr=boolean
  Logical Operator : Logic  AllPortsSameDT=off  OutDataTypeStr=boolean
  Logical Operator1 : Logic  AllPortsSameDT=off  OutDataTypeStr=boolean
  Logical Operator2 : Logic  Operator=OR  AllPortsSameDT=off  OutDataTypeStr=boolean
  Logical Operator3 : Logic  Operator=NOT  AllPortsSameDT=off  OutDataTypeStr=boolean
  Out1 : Outport  VectorParamsAs1DForOutWhenUnconnected=off
  wires:
  In1/1 -> Logical Operator/1
  SEL/1 -> Logical Operator3/1, Logical Operator1/1
  Logical Operator3/1 -> Logical Operator/2
  Logical Operator1/1 -> Logical Operator2/2
  Logical Operator/1 -> Logical Operator2/1
  Logical Operator2/1 -> Out1/1
  In2/1 -> Logical Operator1/2

== system I2S/PISO_SHIFT_REG/MUX3 ==
  note: SEL=0 ==> IN1
  In1 : Inport
  In2 : Inport  Port=2
  SEL : Inport  Port=3  OutDataTypeStr=boolean
  Logical Operator : Logic  AllPortsSameDT=off  OutDataTypeStr=boolean
  Logical Operator1 : Logic  AllPortsSameDT=off  OutDataTypeStr=boolean
  Logical Operator2 : Logic  Operator=OR  AllPortsSameDT=off  OutDataTypeStr=boolean
  Logical Operator3 : Logic  Operator=NOT  AllPortsSameDT=off  OutDataTypeStr=boolean
  Out1 : Outport  VectorParamsAs1DForOutWhenUnconnected=off
  wires:
  In1/1 -> Logical Operator/1
  SEL/1 -> Logical Operator3/1, Logical Operator1/1
  Logical Operator3/1 -> Logical Operator/2
  Logical Operator1/1 -> Logical Operator2/2
  Logical Operator/1 -> Logical Operator2/1
  Logical Operator2/1 -> Out1/1
  In2/1 -> Logical Operator1/2

== system I2S/PISO_SHIFT_REG/MUX30 ==
  note: SEL=0 ==> IN1
  In1 : Inport
  In2 : Inport  Port=2
  SEL : Inport  Port=3  OutDataTypeStr=boolean
  Logical Operator : Logic  AllPortsSameDT=off  OutDataTypeStr=boolean
  Logical Operator1 : Logic  AllPortsSameDT=off  OutDataTypeStr=boolean
  Logical Operator2 : Logic  Operator=OR  AllPortsSameDT=off  OutDataTypeStr=boolean
  Logical Operator3 : Logic  Operator=NOT  AllPortsSameDT=off  OutDataTypeStr=boolean
  Out1 : Outport  VectorParamsAs1DForOutWhenUnconnected=off
  wires:
  In1/1 -> Logical Operator/1
  SEL/1 -> Logical Operator3/1, Logical Operator1/1
  Logical Operator3/1 -> Logical Operator/2
  Logical Operator1/1 -> Logical Operator2/2
  Logical Operator/1 -> Logical Operator2/1
  Logical Operator2/1 -> Out1/1
  In2/1 -> Logical Operator1/2

== system I2S/PISO_SHIFT_REG/MUX31 ==
  note: SEL=0 ==> IN1
  In1 : Inport
  In2 : Inport  Port=2
  SEL : Inport  Port=3  OutDataTypeStr=boolean
  Logical Operator : Logic  AllPortsSameDT=off  OutDataTypeStr=boolean
  Logical Operator1 : Logic  AllPortsSameDT=off  OutDataTypeStr=boolean
  Logical Operator2 : Logic  Operator=OR  AllPortsSameDT=off  OutDataTypeStr=boolean
  Logical Operator3 : Logic  Operator=NOT  AllPortsSameDT=off  OutDataTypeStr=boolean
  Out1 : Outport  VectorParamsAs1DForOutWhenUnconnected=off
  wires:
  In1/1 -> Logical Operator/1
  SEL/1 -> Logical Operator3/1, Logical Operator1/1
  Logical Operator3/1 -> Logical Operator/2
  Logical Operator1/1 -> Logical Operator2/2
  Logical Operator/1 -> Logical Operator2/1
  Logical Operator2/1 -> Out1/1
  In2/1 -> Logical Operator1/2

== system I2S/PISO_SHIFT_REG/MUX4 ==
  note: SEL=0 ==> IN1
  In1 : Inport
  In2 : Inport  Port=2
  SEL : Inport  Port=3  OutDataTypeStr=boolean
  Logical Operator : Logic  AllPortsSameDT=off  OutDataTypeStr=boolean
  Logical Operator1 : Logic  AllPortsSameDT=off  OutDataTypeStr=boolean
  Logical Operator2 : Logic  Operator=OR  AllPortsSameDT=off  OutDataTypeStr=boolean
  Logical Operator3 : Logic  Operator=NOT  AllPortsSameDT=off  OutDataTypeStr=boolean
  Out1 : Outport  VectorParamsAs1DForOutWhenUnconnected=off
  wires:
  In1/1 -> Logical Operator/1
  SEL/1 -> Logical Operator3/1, Logical Operator1/1
  Logical Operator3/1 -> Logical Operator/2
  Logical Operator1/1 -> Logical Operator2/2
  Logical Operator/1 -> Logical Operator2/1
  Logical Operator2/1 -> Out1/1
  In2/1 -> Logical Operator1/2

== system I2S/PISO_SHIFT_REG/MUX5 ==
  note: SEL=0 ==> IN1
  In1 : Inport
  In2 : Inport  Port=2
  SEL : Inport  Port=3  OutDataTypeStr=boolean
  Logical Operator : Logic  AllPortsSameDT=off  OutDataTypeStr=boolean
  Logical Operator1 : Logic  AllPortsSameDT=off  OutDataTypeStr=boolean
  Logical Operator2 : Logic  Operator=OR  AllPortsSameDT=off  OutDataTypeStr=boolean
  Logical Operator3 : Logic  Operator=NOT  AllPortsSameDT=off  OutDataTypeStr=boolean
  Out1 : Outport  VectorParamsAs1DForOutWhenUnconnected=off
  wires:
  In1/1 -> Logical Operator/1
  SEL/1 -> Logical Operator3/1, Logical Operator1/1
  Logical Operator3/1 -> Logical Operator/2
  Logical Operator1/1 -> Logical Operator2/2
  Logical Operator/1 -> Logical Operator2/1
  Logical Operator2/1 -> Out1/1
  In2/1 -> Logical Operator1/2

== system I2S/PISO_SHIFT_REG/MUX6 ==
  note: SEL=0 ==> IN1
  In1 : Inport
  In2 : Inport  Port=2
  SEL : Inport  Port=3  OutDataTypeStr=boolean
  Logical Operator : Logic  AllPortsSameDT=off  OutDataTypeStr=boolean
  Logical Operator1 : Logic  AllPortsSameDT=off  OutDataTypeStr=boolean
  Logical Operator2 : Logic  Operator=OR  AllPortsSameDT=off  OutDataTypeStr=boolean
  Logical Operator3 : Logic  Operator=NOT  AllPortsSameDT=off  OutDataTypeStr=boolean
  Out1 : Outport  VectorParamsAs1DForOutWhenUnconnected=off
  wires:
  In1/1 -> Logical Operator/1
  SEL/1 -> Logical Operator3/1, Logical Operator1/1
  Logical Operator3/1 -> Logical Operator/2
  Logical Operator1/1 -> Logical Operator2/2
  Logical Operator/1 -> Logical Operator2/1
  Logical Operator2/1 -> Out1/1
  In2/1 -> Logical Operator1/2

== system I2S/PISO_SHIFT_REG/MUX7 ==
  note: SEL=0 ==> IN1
  In1 : Inport
  In2 : Inport  Port=2
  SEL : Inport  Port=3  OutDataTypeStr=boolean
  Logical Operator : Logic  AllPortsSameDT=off  OutDataTypeStr=boolean
  Logical Operator1 : Logic  AllPortsSameDT=off  OutDataTypeStr=boolean
  Logical Operator2 : Logic  Operator=OR  AllPortsSameDT=off  OutDataTypeStr=boolean
  Logical Operator3 : Logic  Operator=NOT  AllPortsSameDT=off  OutDataTypeStr=boolean
  Out1 : Outport  VectorParamsAs1DForOutWhenUnconnected=off
  wires:
  In1/1 -> Logical Operator/1
  SEL/1 -> Logical Operator3/1, Logical Operator1/1
  Logical Operator3/1 -> Logical Operator/2
  Logical Operator1/1 -> Logical Operator2/2
  Logical Operator/1 -> Logical Operator2/1
  Logical Operator2/1 -> Out1/1
  In2/1 -> Logical Operator1/2

== system I2S/PISO_SHIFT_REG/MUX8 ==
  note: SEL=0 ==> IN1
  In1 : Inport
  In2 : Inport  Port=2
  SEL : Inport  Port=3  OutDataTypeStr=boolean
  Logical Operator : Logic  AllPortsSameDT=off  OutDataTypeStr=boolean
  Logical Operator1 : Logic  AllPortsSameDT=off  OutDataTypeStr=boolean
  Logical Operator2 : Logic  Operator=OR  AllPortsSameDT=off  OutDataTypeStr=boolean
  Logical Operator3 : Logic  Operator=NOT  AllPortsSameDT=off  OutDataTypeStr=boolean
  Out1 : Outport  VectorParamsAs1DForOutWhenUnconnected=off
  wires:
  In1/1 -> Logical Operator/1
  SEL/1 -> Logical Operator3/1, Logical Operator1/1
  Logical Operator3/1 -> Logical Operator/2
  Logical Operator1/1 -> Logical Operator2/2
  Logical Operator/1 -> Logical Operator2/1
  Logical Operator2/1 -> Out1/1
  In2/1 -> Logical Operator1/2

== system I2S/PISO_SHIFT_REG/MUX9 ==
  note: SEL=0 ==> IN1
  In1 : Inport
  In2 : Inport  Port=2
  SEL : Inport  Port=3  OutDataTypeStr=boolean
  Logical Operator : Logic  AllPortsSameDT=off  OutDataTypeStr=boolean
  Logical Operator1 : Logic  AllPortsSameDT=off  OutDataTypeStr=boolean
  Logical Operator2 : Logic  Operator=OR  AllPortsSameDT=off  OutDataTypeStr=boolean
  Logical Operator3 : Logic  Operator=NOT  AllPortsSameDT=off  OutDataTypeStr=boolean
  Out1 : Outport  VectorParamsAs1DForOutWhenUnconnected=off
  wires:
  In1/1 -> Logical Operator/1
  SEL/1 -> Logical Operator3/1, Logical Operator1/1
  Logical Operator3/1 -> Logical Operator/2
  Logical Operator1/1 -> Logical Operator2/2
  Logical Operator/1 -> Logical Operator2/1
  Logical Operator2/1 -> Out1/1
  In2/1 -> Logical Operator1/2
